simulink subsystem "Outputs_ESP32"  (R2024b)
settings: Solver=VariableStepAuto  StartTime=0.0  StopTime=10.0  RelTol=1e-3
libraries: arduinolib x9
settings Model: Creator=m4ttn  LastModifiedBy=m4ttn

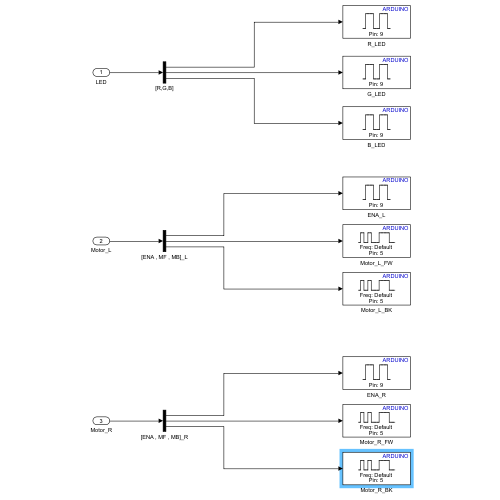
[thumbnail: Simulink's stored preview of the top-level diagram]
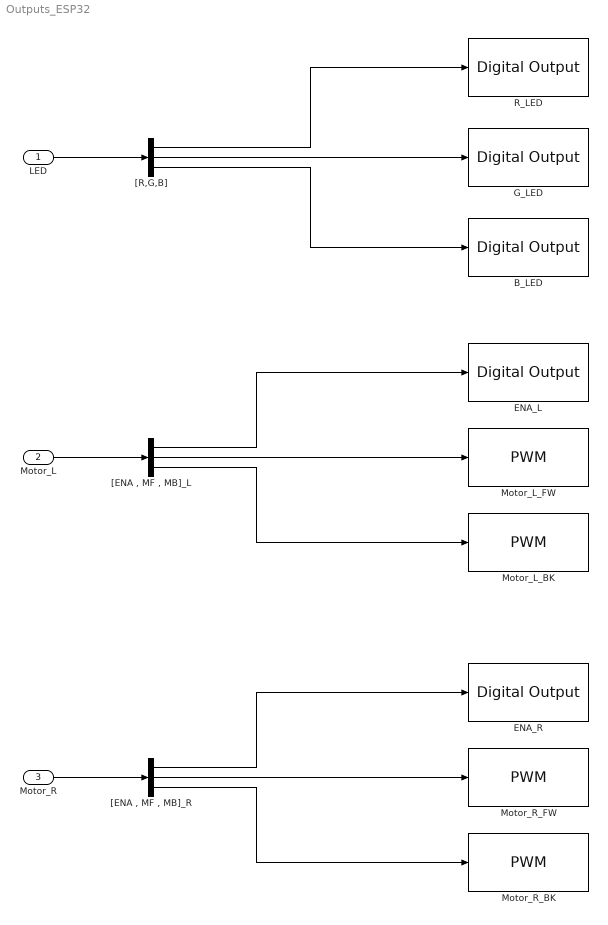
== system Outputs_ESP32 ==
  LED : Inport
  Motor_L : Inport  Port=2
  Motor_R : Inport  Port=3
  B_LED : arduinolib/Digital Output  pinNumber=9  Direction=output  blockPlatform=arduino
  ENA_L : arduinolib/Digital Output  pinNumber=9  Direction=output  blockPlatform=arduino
  ENA_R : arduinolib/Digital Output  pinNumber=9  Direction=output  blockPlatform=arduino
  G_LED : arduinolib/Digital Output  pinNumber=9  Direction=output  blockPlatform=arduino
  Motor_L_BK : arduinolib/PWM  pinNumber=5  frequencyType=Default  desiredFrequency=490.2  achievableFrequency=490.2
  Motor_L_FW : arduinolib/PWM  pinNumber=5  frequencyType=Default  desiredFrequency=490.2  achievableFrequency=490.2
  Motor_R_BK : arduinolib/PWM  pinNumber=5  frequencyType=Default  desiredFrequency=490.2  achievableFrequency=490.2
  Motor_R_FW : arduinolib/PWM  pinNumber=5  frequencyType=Default  desiredFrequency=490.2  achievableFrequency=490.2
  R_LED : arduinolib/Digital Output  pinNumber=9  Direction=output  blockPlatform=arduino
  "[ENA , MF , MB]_L" : Demux  Outputs=3
  "[ENA , MF , MB]_R" : Demux  Outputs=3
  "[R,G,B]" : Demux  Outputs=3
  wires:
  LED/1 -> "[R,G,B]"/1
  "[R,G,B]"/1 -> R_LED/1
  "[R,G,B]"/2 -> G_LED/1
  "[R,G,B]"/3 -> B_LED/1
  Motor_L/1 -> "[ENA , MF , MB]_L"/1
  "[ENA , MF , MB]_L"/1 -> ENA_L/1
  "[ENA , MF , MB]_L"/2 -> Motor_L_FW/1
  "[ENA , MF , MB]_L"/3 -> Motor_L_BK/1
  Motor_R/1 -> "[ENA , MF , MB]_R"/1
  "[ENA , MF , MB]_R"/3 -> Motor_R_BK/1
  "[ENA , MF , MB]_R"/1 -> ENA_R/1
  "[ENA , MF , MB]_R"/2 -> Motor_R_FW/1
